simulink model "evaluateParamVar"  (Simulink 7.4)
settings: Solver=ode45  SolverMode=SingleTasking  StartTime=0.0  StopTime=0.4  RelTol=1e-3
values from neighbouring files (symbols this model uses):
  plant = tf(1,[0.01 1])    [transferfunDisObserver_sim.m]
  plantWithVar = plant*1/1.5    [transferfunDisObserver_sim.m]
settings Model: Creator=Yu  LastModifiedBy=Yu  CovMetricSettings=dwe  CovHtmlReporting=off  covSaveCumulativeToWorkspaceVar=off  CovSaveSingleToWorkspaceVar=off  CovExternalEMLEnable=on
settings DataIOCC: LimitDataPoints=off  SaveFormat=StructureWithTime
settings OptimizationCC: ExpressionDepthLimit=128
settings DebuggingCC: UnderspecifiedInitializationDetection=Simplified  MergeDetectMultiDrivingBlocksExec=error  SolverPrmCheckMsg=none  FcnCallInpInsideContextMsg=Enable All  StateNameClashWarn=none  StrictBusMsg=ErrorLevel1
settings HardwareCC: ProdIntDivRoundTo=Zero  ProdEndianess=LittleEndian  ProdHWDeviceType=Specified
settings CodeAppCC: CustomSymbolStrType=$N$R$M_T
settings GRTTargetCC: TargetFunctionLibrary=C99 (ISO)  GeneratePreprocessorConditionals=Use local settings

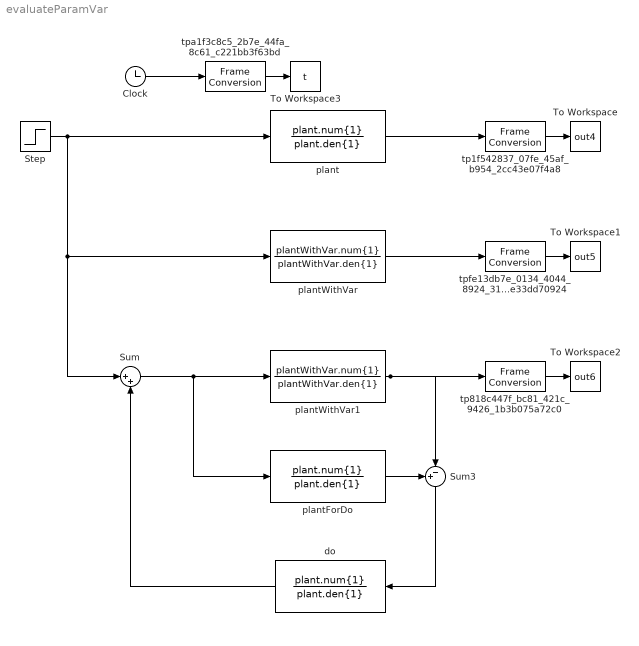
== system evaluateParamVar ==
  Clock : Clock
  Step : Step  Time=0.01  SampleTime=0
  Sum : Sum  Inputs=|++
  Sum3 : Sum  Inputs=+-|
  To Workspace : ToWorkspace  VariableName=out4  SampleTime=-1
  To Workspace1 : ToWorkspace  VariableName=out5  SampleTime=-1
  To Workspace2 : ToWorkspace  VariableName=out6  SampleTime=-1
  To Workspace3 : ToWorkspace  VariableName=t  SampleTime=-1
  do : TransferFcn  Numerator=plant.num{1}  Denominator=plant.den{1}
  plant : TransferFcn  Numerator=plant.num{1}  Denominator=plant.den{1}
  plantForDo : TransferFcn  Numerator=plant.num{1}  Denominator=plant.den{1}
  plantWithVar : TransferFcn  Numerator=plantWithVar.num{1}  Denominator=plantWithVar.den{1}
  plantWithVar1 : TransferFcn  Numerator=plantWithVar.num{1}  Denominator=plantWithVar.den{1}
  tp1f542837_07fe_45af_b954_2cc43e07f4a8 : FrameConversion  InheritSamplingMode=off  OutFrame=Sample-based
  tp818c447f_bc81_421c_9426_1b3b075a72c0 : FrameConversion  InheritSamplingMode=off  OutFrame=Sample-based
  tpa1f3c8c5_2b7e_44fa_8c61_c221bb3f63bd : FrameConversion  InheritSamplingMode=off  OutFrame=Sample-based
  tpfe13db7e_0134_4044_8924_31e33dd70924 : FrameConversion  InheritSamplingMode=off  OutFrame=Sample-based
  wires:
  Step/1 -> plant/1, Sum/1, plantWithVar/1
  Sum/1 -> plantForDo/1, plantWithVar1/1
  do/1 -> Sum/2
  plantWithVar1/1 -> Sum3/2, tp818c447f_bc81_421c_9426_1b3b075a72c0/1
  plantForDo/1 -> Sum3/1
  Sum3/1 -> do/1
  plant/1 -> tp1f542837_07fe_45af_b954_2cc43e07f4a8/1
  tp1f542837_07fe_45af_b954_2cc43e07f4a8/1 -> To Workspace/1
  plantWithVar/1 -> tpfe13db7e_0134_4044_8924_31e33dd70924/1
  tpfe13db7e_0134_4044_8924_31e33dd70924/1 -> To Workspace1/1
  tp818c447f_bc81_421c_9426_1b3b075a72c0/1 -> To Workspace2/1
  Clock/1 -> tpa1f3c8c5_2b7e_44fa_8c61_c221bb3f63bd/1
  tpa1f3c8c5_2b7e_44fa_8c61_c221bb3f63bd/1 -> To Workspace3/1
